simulink model "isentropic_nozzle"  (R2024b)
settings: Solver=VariableStepAuto  StartTime=0.0  StopTime=10.0  RelTol=1e-3
libraries: fl_lib x7, nesl_utility x5
(part 2 of 2)

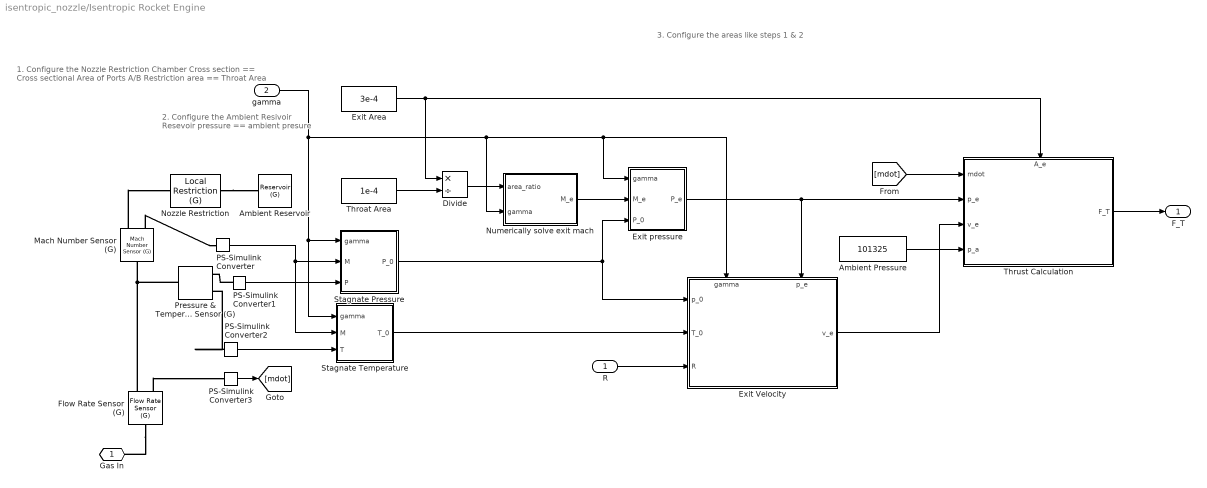
== system isentropic_nozzle/Isentropic Rocket Engine ==
  note: 2. Configure the Ambient Resivoir
      | Resevoir pressure == ambient presure
  note: 3. Configure the areas like steps 1 & 2
  note: 1. Configure the Nozzle Restriction
      | Chamber Cross section == Cross sectional Area of Ports A/B
      | Restriction area == Throat Area
  R : Inport
  gamma : Inport  Port=2
  Ambient Pressure : Constant  Value=101325
  Ambient Reservoir : fl_lib/Gas/Elements/Reservoir (G)  pressure_spec=foundation.enum.pressure_spec.specified  reservoir_pressure=0.101325 MPa  reservoir_temperature=300 K  area_A=3e-4 m^2
  Divide : Product  Inputs=*/
  Exit Area : Constant  Value=3e-4
  Exit Velocity : Subsystem
      settings: PortSchema="{\"entries\":[{\"content\":{\"sides\":[{\"content\":{\"connectorIds\":[\"In1\",\"In2\",\"In3\"]},\"type\":\"ConnectorPlacement.EquallySpacedRectSide\",\"uuid\":\"9662f2ce-6bfa-421c-bf6e-2b5a914169e1\"},{\"content\":{\"connectorIds\":[\"Out1\"],\"side\":\"RIGHT\"},\"type\":\"ConnectorPlacement.EquallySpacedRectSide\",\"uuid\":\"c1c18a70-1766-4293-aa61-9a3b121d2f3e\"},{\"content\":{\"connectorIds\":[\"In4\",\"In5\"],\"side\":\"TOP\"},\"type\":\"ConnectorPlacement.EquallySpacedRectSide\",\"uuid\":\"849a73b4-5870-485a-955e-1c277ed91a42\"}]},\"type\":\"ConnectorPlacement.EquallySpacedConnector\",\"uuid\":\"ef3d261f-478e-436f-9ab2-12f2688af38d\"}],\"packageUris\":[\"http://schema.mathworks.com/mf0/Connector/R2020b\"],\"version\":\"1.0\"}"
  Exit pressure : Subsystem
  Flow Rate Sensor (G) : fl_lib/Gas/Sensors/Flow Rate Sensor (G)  mass_flow_measure=true  volumetric_flow_measure=false  volumetric_flow_conditions=foundation.enum.volumetric_flow_conditions.actual  p_std=0.101325 MPa  T_std=20 degC  energy_flow_measure=false
      settings: InternalSimscapePortConfiguration="{\"Bottom\":[],\"Left\":[{\"id\":\"A\",\"label\":\"A\",\"type\":\"foundation.gas.gas\"}],\"Right\":[{\"id\":\"B\",\"label\":\"B\",\"type\":\"foundation.gas.gas\"},{\"id\":\"M\",\"label\":\"M\",\"type\":\"output\"}],\"Top\":[]}"
  Mach Number Sensor (G) : fl_lib/Gas/Sensors/Mach Number Sensor (G)  area=0.01 m^2
      settings: InternalSimscapePortConfiguration="{\"Bottom\":[{\"id\":\"Mach\",\"label\":\"Mach\",\"type\":\"output\"}],\"Left\":[{\"id\":\"A\",\"label\":\"A\",\"type\":\"foundation.gas.gas\"}],\"Right\":[{\"id\":\"B\",\"label\":\"B\",\"type\":\"foundation.gas.gas\"}],\"Top\":[]}"
  Nozzle Restriction : fl_lib/Gas/Elements/Local Restriction (G)  restriction_type=foundation.enum.restriction_type.fixed  restriction_area=1e-4 m^2  min_area=1e-10 m^2  max_area=0.005 m^2  area=2e-4 m^2  Cd=1.0  B_lam=0.999
      settings: InternalSimscapePortConfiguration="{\"Bottom\":[],\"Left\":[{\"id\":\"A\",\"label\":\"A\",\"type\":\"foundation.gas.gas\"}],\"Right\":[{\"id\":\"B\",\"label\":\"B\",\"type\":\"foundation.gas.gas\"}],\"Top\":[]}"
  Numerically solve exit mach : MATLAB Function  TreatAsAtomicUnit=on
  PS-Simulink Converter{,1..3} (4 alike) : nesl_utility/PS-Simulink Converter  PhysicalDomain=network_engine_domain  SubClassName=ps_output  LeftPortType=input  RightPortType=output  PseudoPeriodic=off  Frequencies=[]  VectorFormat=inherit  Unit=inherit  AffineConversion=off
  Pressure & Temperature Sensor (G) : fl_lib/Gas/Sensors/Pressure & Temperature Sensor (G)  reference=foundation.enum.MeasurementReference.absolute  pressure=true  pressure_spec=foundation.enum.PressureMeasementSpec.Absolute  temperature=true
      settings: InternalSimscapePortConfiguration="{\"Bottom\":[{\"id\":\"T\",\"label\":\"T\",\"type\":\"output\"}],\"Left\":[{\"id\":\"A\",\"label\":\"A\",\"type\":\"foundation.gas.gas\"}],\"Right\":[{\"id\":\"Pa\",\"label\":\"Pa\",\"type\":\"output\"}],\"Top\":[]}"
  Stagnate Pressure : Subsystem
  Stagnate Temperature : Subsystem
  Throat Area : Constant  Value=1e-4
  Thrust Calculation : Subsystem
      settings: PortSchema="{\"entries\":[{\"content\":{\"sides\":[{\"content\":{\"connectorIds\":[\"In1\",\"In2\",\"In3\",\"In4\"]},\"type\":\"ConnectorPlacement.EquallySpacedRectSide\",\"uuid\":\"9662f2ce-6bfa-421c-bf6e-2b5a914169e1\"},{\"content\":{\"connectorIds\":[\"Out1\"],\"side\":\"RIGHT\"},\"type\":\"ConnectorPlacement.EquallySpacedRectSide\",\"uuid\":\"c1c18a70-1766-4293-aa61-9a3b121d2f3e\"},{\"content\":{\"connectorIds\":[\"In5\"],\"side\":\"TOP\"},\"type\":\"ConnectorPlacement.EquallySpacedRectSide\",\"uuid\":\"849a73b4-5870-485a-955e-1c277ed91a42\"}]},\"type\":\"ConnectorPlacement.EquallySpacedConnector\",\"uuid\":\"ef3d261f-478e-436f-9ab2-12f2688af38d\"}],\"packageUris\":[\"http://schema.mathworks.com/mf0/Connector/R2020b\"],\"version\":\"1.0\"}"
  Gas In : PMIOPort  Side=Left
  F_T : Outport
  wires:
  Exit Velocity/1(v_e) -> Thrust Calculation/3(v_e)
  Numerically solve exit mach/1(M_e) -> Exit pressure/2(M_e)
  Stagnate Pressure/1(P_0) -> Exit Velocity/1(p_0), Exit pressure/3(P_0)
  PS-Simulink Converter3/1 -> [mdot]
  Exit Area/1 -> Thrust Calculation/5(A_e), Divide/1
  Throat Area/1 -> Divide/2
  gamma/1 -> Numerically solve exit mach/2(gamma), Exit Velocity/4(gamma), Exit pressure/1(gamma), Stagnate Temperature/1(gamma), Stagnate Pressure/1(gamma)
  Thrust Calculation/1(F_T) -> F_T/1
  [mdot] -> Thrust Calculation/1(mdot)
  Exit pressure/1(P_e) -> Exit Velocity/5(p_e), Thrust Calculation/2(p_e)
  PS-Simulink Converter/1 -> Stagnate Temperature/2(M), Stagnate Pressure/2(M)
  PS-Simulink Converter2/1 -> Stagnate Temperature/3(T)
  R/1 -> Exit Velocity/3(R)
  Ambient Pressure/1 -> Thrust Calculation/4(p_a)
  Stagnate Temperature/1(T_0) -> Exit Velocity/2(T_0)
  Divide/1 -> Numerically solve exit mach/1(area_ratio)
  PS-Simulink Converter1/1 -> Stagnate Pressure/3(P)
  connections:
  Nozzle Restriction/RConn1 -- Ambient Reservoir/LConn1
  PS-Simulink Converter1/LConn1 -- Pressure & Temperature Sensor (G)/RConn1
  Flow Rate Sensor (G)/RConn1 -- Pressure & Temperature Sensor (G)/LConn1 -- Mach Number Sensor (G)/LConn1
  Mach Number Sensor (G)/RConn1 -- Nozzle Restriction/LConn1
  Mach Number Sensor (G)/RConn2 -- PS-Simulink Converter/LConn1
  PS-Simulink Converter2/LConn1 -- Pressure & Temperature Sensor (G)/RConn2
  Flow Rate Sensor (G)/RConn2 -- PS-Simulink Converter3/LConn1
  Flow Rate Sensor (G)/LConn1 -- Gas In/RConn1

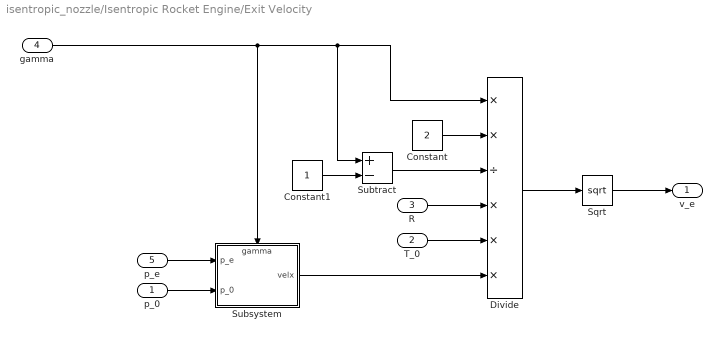
== system isentropic_nozzle/Isentropic Rocket Engine/Exit Velocity ==
  p_0 : Inport
  T_0 : Inport  Port=2
  R : Inport  Port=3
  gamma : Inport  Port=4
  p_e : Inport  Port=5
  Constant : Constant  Value=2
  Constant1 : Constant
  Divide : Product  Inputs=**/***
  Sqrt : Sqrt
  Subsystem : Subsystem
      settings: PortSchema="{\"entries\":[{\"content\":{\"sides\":[{\"content\":{\"connectorIds\":[\"In1\",\"In2\"]},\"type\":\"ConnectorPlacement.EquallySpacedRectSide\",\"uuid\":\"80528716-0a09-4b76-bb3b-dedd14436ef6\"},{\"content\":{\"connectorIds\":[\"Out1\"],\"side\":\"RIGHT\"},\"type\":\"ConnectorPlacement.EquallySpacedRectSide\",\"uuid\":\"42bd620c-9479-4472-9344-ba1c598547ab\"},{\"content\":{\"connectorIds\":[\"In3\"],\"side\":\"TOP\"},\"type\":\"ConnectorPlacement.EquallySpacedRectSide\",\"uuid\":\"08b90db1-f4c9-419f-85b7-12c7462735bc\"}]},\"type\":\"ConnectorPlacement.EquallySpacedConnector\",\"uuid\":\"33a35b9a-f450-40d1-a1fa-c9836b5a81da\"}],\"packageUris\":[\"http://schema.mathworks.com/mf0/Connector/R2020b\"],\"version\":\"1.0\"}"
  Subtract : Sum  Inputs=+-
  v_e : Outport
  wires:
  gamma/1 -> Subtract/1, Divide/1, Subsystem/3(gamma)
  Constant/1 -> Divide/2
  Constant1/1 -> Subtract/2
  Subtract/1 -> Divide/3
  R/1 -> Divide/4
  T_0/1 -> Divide/5
  Divide/1 -> Sqrt/1
  Sqrt/1 -> v_e/1
  Subsystem/1(velx) -> Divide/6
  p_e/1 -> Subsystem/1(p_e)
  p_0/1 -> Subsystem/2(p_0)

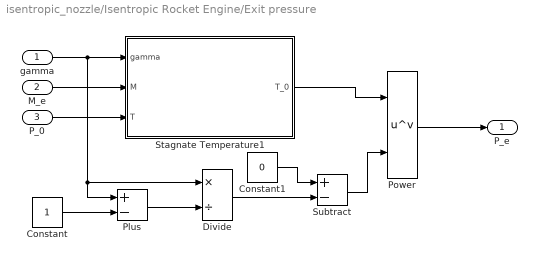
== system isentropic_nozzle/Isentropic Rocket Engine/Exit pressure ==
  gamma : Inport
  M_e : Inport  Port=2
  P_0 : Inport  Port=3
  Constant : Constant
  Constant1 : Constant  Value=0
  Divide : Product  Inputs=*/
  Plus : Sum  Inputs=+-
  Power : Math  Operator=pow
  Stagnate Temperature1 : Subsystem
  Subtract : Sum  Inputs=+-
  P_e : Outport
  wires:
  Constant/1 -> Plus/2
  Plus/1 -> Divide/2
  Power/1 -> P_e/1
  gamma/1 -> Stagnate Temperature1/1(gamma), Plus/1, Divide/1
  P_0/1 -> Stagnate Temperature1/3(T)
  Stagnate Temperature1/1(T_0) -> Power/1
  M_e/1 -> Stagnate Temperature1/2(M)
  Divide/1 -> Subtract/2
  Constant1/1 -> Subtract/1
  Subtract/1 -> Power/2

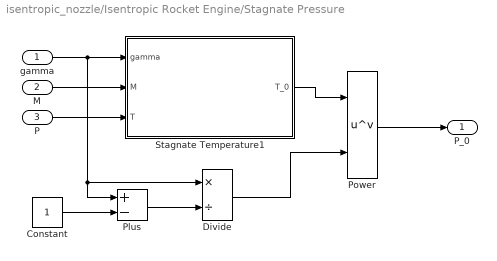
== system isentropic_nozzle/Isentropic Rocket Engine/Stagnate Pressure ==
  gamma : Inport
  M : Inport  Port=2
  P : Inport  Port=3
  Constant : Constant
  Divide : Product  Inputs=*/
  Plus : Sum  Inputs=+-
  Power : Math  Operator=pow
  Stagnate Temperature1 : Subsystem
  P_0 : Outport
  wires:
  M/1 -> Stagnate Temperature1/2(M)
  Stagnate Temperature1/1(T_0) -> Power/1
  P/1 -> Stagnate Temperature1/3(T)
  gamma/1 -> Divide/1, Plus/1, Stagnate Temperature1/1(gamma)
  Divide/1 -> Power/2
  Power/1 -> P_0/1
  Plus/1 -> Divide/2
  Constant/1 -> Plus/2

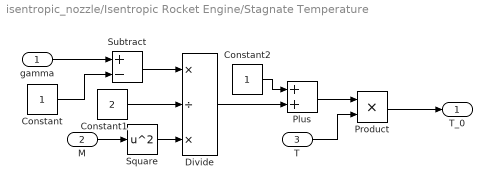
== system isentropic_nozzle/Isentropic Rocket Engine/Stagnate Temperature ==
  gamma : Inport
  M : Inport  Port=2
  T : Inport  Port=3
  Constant : Constant
  Constant1 : Constant  Value=2
  Constant2 : Constant
  Divide : Product  Inputs=*/*
  Plus : Sum
  Product : Product
  Square : Math  Operator=square
  Subtract : Sum  Inputs=+-
  T_0 : Outport
  wires:
  Subtract/1 -> Divide/1
  Constant1/1 -> Divide/2
  gamma/1 -> Subtract/1
  T/1 -> Product/2
  M/1 -> Square/1
  Divide/1 -> Plus/2
  Constant/1 -> Subtract/2
  Constant2/1 -> Plus/1
  Product/1 -> T_0/1
  Square/1 -> Divide/3
  Plus/1 -> Product/1

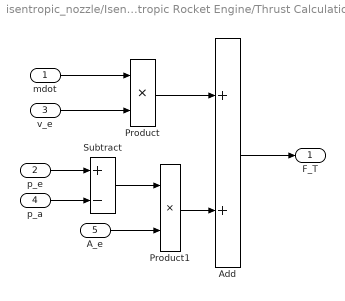
== system isentropic_nozzle/Isentropic Rocket Engine/Thrust Calculation ==
  mdot : Inport
  p_e : Inport  Port=2
  v_e : Inport  Port=3
  p_a : Inport  Port=4
  A_e : Inport  Port=5
  Add : Sum
  Product : Product
  Product1 : Product
  Subtract : Sum  Inputs=+-
  F_T : Outport
  wires:
  Subtract/1 -> Product1/1
  Product/1 -> Add/1
  A_e/1 -> Product1/2
  p_a/1 -> Subtract/2
  Add/1 -> F_T/1
  mdot/1 -> Product/1
  Product1/1 -> Add/2
  p_e/1 -> Subtract/1
  v_e/1 -> Product/2

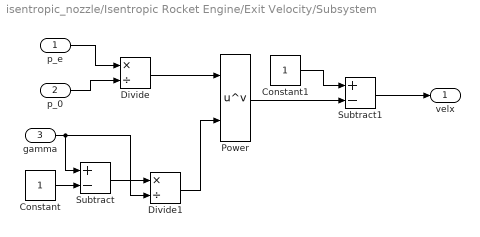
== system isentropic_nozzle/Isentropic Rocket Engine/Exit Velocity/Subsystem ==
  p_e : Inport
  p_0 : Inport  Port=2
  gamma : Inport  Port=3
  Constant : Constant
  Constant1 : Constant
  Divide : Product  Inputs=*/
  Divide1 : Product  Inputs=*/
  Power : Math  Operator=pow
  Subtract : Sum  Inputs=+-
  Subtract1 : Sum  Inputs=+-
  velx : Outport
  wires:
  p_e/1 -> Divide/1
  p_0/1 -> Divide/2
  Divide/1 -> Power/1
  gamma/1 -> Divide1/2, Subtract/1
  Constant/1 -> Subtract/2
  Subtract/1 -> Divide1/1
  Divide1/1 -> Power/2
  Power/1 -> Subtract1/2
  Constant1/1 -> Subtract1/1
  Subtract1/1 -> velx/1

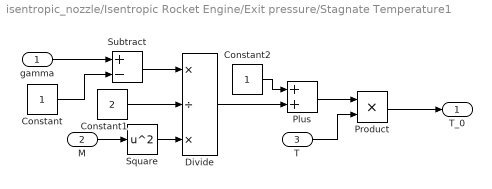
== system isentropic_nozzle/Isentropic Rocket Engine/Exit pressure/Stagnate Temperature1 ==
  gamma : Inport
  M : Inport  Port=2
  T : Inport  Port=3
  Constant : Constant
  Constant1 : Constant  Value=2
  Constant2 : Constant
  Divide : Product  Inputs=*/*
  Plus : Sum
  Product : Product
  Square : Math  Operator=square
  Subtract : Sum  Inputs=+-
  T_0 : Outport
  wires:
  Subtract/1 -> Divide/1
  Constant1/1 -> Divide/2
  gamma/1 -> Subtract/1
  T/1 -> Product/2
  M/1 -> Square/1
  Divide/1 -> Plus/2
  Constant/1 -> Subtract/2
  Constant2/1 -> Plus/1
  Product/1 -> T_0/1
  Square/1 -> Divide/3
  Plus/1 -> Product/1

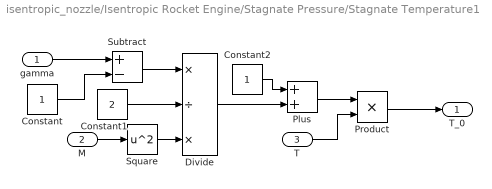
== system isentropic_nozzle/Isentropic Rocket Engine/Stagnate Pressure/Stagnate Temperature1 ==
  gamma : Inport
  M : Inport  Port=2
  T : Inport  Port=3
  Constant : Constant
  Constant1 : Constant  Value=2
  Constant2 : Constant
  Divide : Product  Inputs=*/*
  Plus : Sum
  Product : Product
  Square : Math  Operator=square
  Subtract : Sum  Inputs=+-
  T_0 : Outport
  wires:
  Plus/1 -> Product/1
  Square/1 -> Divide/3
  Product/1 -> T_0/1
  Constant2/1 -> Plus/1
  Constant/1 -> Subtract/2
  Divide/1 -> Plus/2
  M/1 -> Square/1
  T/1 -> Product/2
  gamma/1 -> Subtract/1
  Constant1/1 -> Divide/2
  Subtract/1 -> Divide/1

== matlab function isentropic_nozzle/Isentropic Rocket Engine/Numerically solve exit mach ==
  data: area_ratio input; M_e output; gamma input
function M_e = fn(area_ratio, gamma)
% Solve the area-Mach relation numerically

    f = @(M) (1./M) .* ...
        ( (2/(gamma+1)) * (1 + (gamma-1)/2 * M.^2) ).^((gamma+1)/(2*(gamma-1))) ...
        - area_ratio;

    % Guess supersonic
    M_e = fzero(f, [1.01 10]);
end
